simulink model "Jaco_3_7_IK"  (R2017a)
settings: Solver=VariableStepAuto  StartTime=0.0  StopTime=10.0  RelTol=1e-3  EnableMultiTasking=on
libraries: mblibv1 x42
settings Model: Creator=litia  LastModifiedBy=nathalie
settings OptimizationCC: LifeSpan=inf
settings DebuggingCC: SFUnexpectedBacktrackingDiag=warning  SFNoUnconditionalDefaultTransitionDiag=warning  SFExecutionAtInitializationDiag=none
settings GRTTargetCC: TargetLangStandard=C89/C90 (ANSI)
settings ConfigComp: CovMetricSettings=dw  CovHtmlReporting=on  CovSaveCumulativeToWorkspaceVar=on  CovSaveSingleToWorkspaceVar=on  CovExternalEMLEnable=off
settings SimMechanicsCC: VisOnUpdateDiagram=on  VisDuringSimulation=on

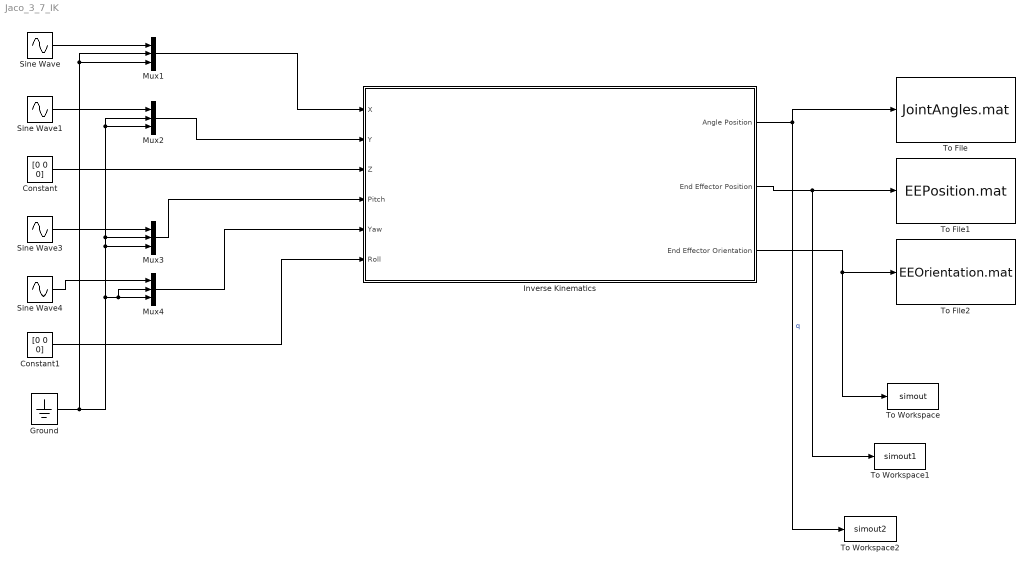
== system Jaco_3_7_IK ==
  Constant : Constant  Value=[0 0 0]  VectorParams1D=off
  Constant1 : Constant  Value=[0 0 0]  VectorParams1D=off
  Ground : Ground
  "Inverse Kinematics " : Subsystem
  Mux{1..4} (4 alike) : Mux  Inputs=3
  Sine Wave : Sin  Amplitude=0.2  Bias=-2  Frequency=2*pi  Phase=pi/2  SampleTime=0
  Sine Wave1 : Sin  Amplitude=0.2  Bias=-1  Frequency=2*pi  SampleTime=0
  Sine Wave3 : Sin  Amplitude=10  Bias=85  Frequency=2*pi  Phase=pi  SampleTime=0
  Sine Wave4 : Sin  Amplitude=10  Frequency=2*pi  Phase=pi/2  SampleTime=0
  To File : ToFile  Filename=JointAngles.mat  MatrixName=q  SaveFormat=Timeseries
  To File1 : ToFile  Filename=EEPosition.mat  MatrixName=xe  SaveFormat=Timeseries
  To File2 : ToFile  Filename=EEOrientation.mat  MatrixName=thetae  SaveFormat=Timeseries
  To Workspace : ToWorkspace  VariableName=simout  SaveFormat=Timeseries  SampleTime=-1
  To Workspace1 : ToWorkspace  VariableName=simout1  SaveFormat=Timeseries  SampleTime=-1
  To Workspace2 : ToWorkspace  VariableName=simout2  SaveFormat=Timeseries  SampleTime=-1
  wires:
  "Inverse Kinematics "/1("Angle Position ") -> To File/1, To Workspace2/1  "q"
  "Inverse Kinematics "/2(End Effector Position) -> To Workspace1/1, To File1/1
  "Inverse Kinematics "/3(End Effector Orientation) -> To Workspace/1, To File2/1
  Sine Wave/1 -> Mux1/1
  Sine Wave1/1 -> Mux2/1
  Ground/1 -> Mux1/3, Mux1/2, Mux3/3, Mux3/2, Mux2/3, Mux2/2, Mux4/2, Mux4/3
  Mux3/1 -> "Inverse Kinematics "/4(Pitch)
  Mux4/1 -> "Inverse Kinematics "/5(Yaw)
  Mux1/1 -> "Inverse Kinematics "/1(" X")
  Mux2/1 -> "Inverse Kinematics "/2(Y)
  Constant1/1 -> "Inverse Kinematics "/6("Roll ")
  Constant/1 -> "Inverse Kinematics "/3(Z)
  Sine Wave3/1 -> Mux3/1
  Sine Wave4/1 -> Mux4/1

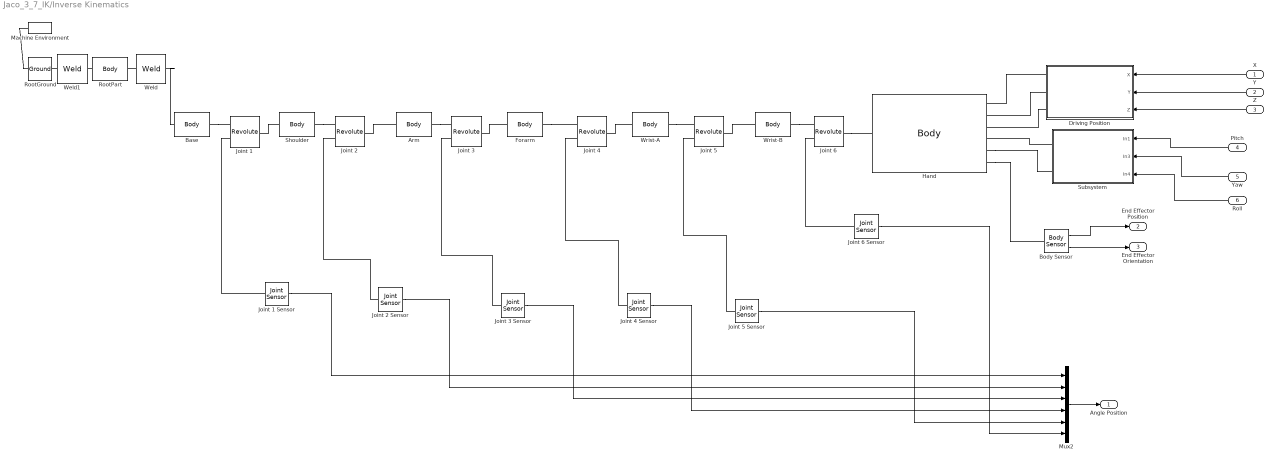
== system Jaco_3_7_IK/Inverse Kinematics  ==
  " X" : Inport
  Y : Inport  Port=2
  Z : Inport  Port=3
  Pitch : Inport  Port=4
  Yaw : Inport  Port=5
  "Roll " : Inport  Port=6
  Arm : mblibv1/Bodies/Body  LConnTagsString=CS2  RConnTagsString=CS3  UpdateFromCAD=on  DialogClass=MechanicalBodyBlock  Mass=1.056  MassUnits=kg  InertiaUnits=kg*m^2  Inertia=[0.0375645,-1.33324e-07,0.000108785;-1.33324e-07,0.0372402,-2.39225e-07;0.000108785,-2.39225e-07,0.00059301]  Shape=Cylinder  ShapeDims=[1 1]  ShapeUnits=m  ShapeUse=false  Density=1  DensityUnits=kg/m^3  DensityUse=false  GraphicsMode=GFXFILE  GraphicsFileName=Jaco_3_7 - arm_ass-1.STL  BodyColorSelMode=COLORPALETTE  BodyColor=[0.752941;0.752941;0.752941]  AttachedToCS=CS1  CG=Right$CG$[0.10282 0.0944444 0.508793]$WORLD$WORLD$m$[0.695251 0.715707 -0.0662524;0.718767 -0.692291 0.0640847;0 -0.092175 -0.995743]$3x3 Transform$rad$WORLD$false$none  WorkingFrames=Right$CS1$[-0.183907 0.105598 0.903425]$WORLD$WORLD$m$[0.695251 0.715707 -0.0662524;0.718767 -0.692291 0.0640847;0 -0.092175 -0.995743]$3x3 Transform$rad$WORLD$false$none#Left$CS2$[0.0767642 0.095252 0.300589]$WORLD$WORLD$m$[1 0 0;0 1 0;0 0 1]$3x3 Transform$rad$WORLD$true$none#Right$CS3$[0.10358 0.0686179 0.708843]$WORLD$WORLD$m$[1 0 0;0 1 0;0 0 1]$3x3 Transform$rad$WORLD$true$none  CGPos=[0.10282 0.0944444 0.508793]  CGRot=[0.695251 0.715707 -0.0662524;0.718767 -0.692291 0.0640847;0 -0.092175 -0.995743]  CS0Pos=[]  CS0Rot=[]  CS1Pos=[-0.183907 0.105598 0.903425]  CS1Rot=[0.695251 0.715707 -0.0662524;0.718767 -0.692291 0.0640847;0 -0.092175 -0.995743]  CS2Pos=[0.0767642 0.095252 0.300589]  CS2Rot=[1 0 0;0 1 0;0 0 1]  CS3Pos=[0.10358 0.0686179 0.708843]  CS3Rot=[1 0 0;0 1 0;0 0 1]  CS4Pos=[]  CS4Rot=[]  CS5Pos=[]  CS5Rot=[]  CS6Pos=[]  CS6Rot=[]  CS7Pos=[]  CS7Rot=[]  CS8Pos=[]  CS8Rot=[]  CS9Pos=[]  CS9Rot=[]  CS10Pos=[]  CS10Rot=[]  CS11Pos=[]  CS11Rot=[]  CS12Pos=[]  CS12Rot=[]  CS13Pos=[]  CS13Rot=[]  CS14Pos=[]  CS14Rot=[]  CS15Pos=[]  CS15Rot=[]  CS16Pos=[]  CS16Rot=[]  CS17Pos=[]  CS17Rot=[]  CS18Pos=[]  CS18Rot=[]  CS19Pos=[]  CS19Rot=[]  CS20Pos=[]  CS20Rot=[]
      settings: SourceProductName=Simscape Multibody  SourceProductBaseCode=MS
  Base : mblibv1/Bodies/Body  LConnTagsString=CS2  RConnTagsString=CS3  UpdateFromCAD=on  DialogClass=MechanicalBodyBlock  Mass=0.570939  MassUnits=kg  InertiaUnits=kg*m^2  Inertia=[0.00175947,1.92772e-07,-3.1782e-05;1.92772e-07,0.00176256,-3.18122e-05;-3.1782e-05,-3.18122e-05,0.000478232]  Shape=Cylinder  ShapeDims=[1 1]  ShapeUnits=m  ShapeUse=false  Density=1  DensityUnits=kg/m^3  DensityUse=false  GraphicsMode=GFXFILE  GraphicsFileName=Jaco_3_7 - base_ass-1.STL  BodyColorSelMode=COLORPALETTE  BodyColor=[0.752941;0.752941;0.752941]  AttachedToCS=CS1  CG=Right$CG$[0.0747134 0.093124 0.128067]$WORLD$WORLD$m$[1 0 0;0 1 0;0 0 1]$3x3 Transform$rad$WORLD$false$none  WorkingFrames=Right$CS1$[0.106448 0.0299726 -0.0762042]$WORLD$WORLD$m$[1 0 0;0 1 0;0 0 1]$3x3 Transform$rad$WORLD$false$none#Left$CS2$[0.0747134 0.093124 0.128067]$WORLD$WORLD$m$[1 0 0;0 1 0;0 0 1]$3x3 Transform$rad$WORLD$true$none#Right$CS3$[0.0753736 0.0938145 0.182089]$WORLD$WORLD$m$[1 0 0;0 1 0;0 0 1]$3x3 Transform$rad$WORLD$true$none  CGPos=[0.0747134 0.093124 0.128067]  CGRot=[1 0 0;0 1 0;0 0 1]  CS0Pos=[]  CS0Rot=[]  CS1Pos=[0.106448 0.0299726 -0.0762042]  CS1Rot=[1 0 0;0 1 0;0 0 1]  CS2Pos=[0.0747134 0.093124 0.128067]  CS2Rot=[1 0 0;0 1 0;0 0 1]  CS3Pos=[0.0753736 0.0938145 0.182089]  CS3Rot=[1 0 0;0 1 0;0 0 1]  CS4Pos=[]  CS4Rot=[]  CS5Pos=[]  CS5Rot=[]  CS6Pos=[]  CS6Rot=[]  CS7Pos=[]  CS7Rot=[]  CS8Pos=[]  CS8Rot=[]  CS9Pos=[]  CS9Rot=[]  CS10Pos=[]  CS10Rot=[]  CS11Pos=[]  CS11Rot=[]  CS12Pos=[]  CS12Rot=[]  CS13Pos=[]  CS13Rot=[]  CS14Pos=[]  CS14Rot=[]  CS15Pos=[]  CS15Rot=[]  CS16Pos=[]  CS16Rot=[]  CS17Pos=[]  CS17Rot=[]  CS18Pos=[]  CS18Rot=[]  CS19Pos=[]  CS19Rot=[]  CS20Pos=[]  CS20Rot=[]
      settings: SourceProductName=Simscape Multibody  SourceProductBaseCode=MS
  Body Sensor : mblibv1/Sensors &  Actuators/Body Sensor  UpdateFromCAD=off  PhysicalDomain=Mechanical  PortType=blob  Muxed=off  Pose=on  Angle=on  AngleUnits=deg  ArcVelocity=off  ArcVelocityUnits=deg/s  ArcAcceleration=off  ArcAccelerationUnits=deg/s^2  CoordPosition=on  CoordPositionUnits=m  Velocity=off  VelocityUnits=m/s  Acceleration=off  AccelerationUnits=m/s^2  Quaternion=on  QuaternionDT=off  QuaternionDDT=off  QuaternionUnits=off  OutputVector=[1]  ActiveIO=on  Width=12  DialogClass=MechanicalSensorBlock  ReferenceFrame=Absolute (World)
      settings: SourceProductName=Simscape Multibody  SourceProductBaseCode=MS
  Driving Position : Subsystem
  Forarm : mblibv1/Bodies/Body  LConnTagsString=CS2  RConnTagsString=CS3  UpdateFromCAD=on  DialogClass=MechanicalBodyBlock  Mass=0.735414  MassUnits=kg  InertiaUnits=kg*m^2  Inertia=[0.00626271,-0.000115651,1.81814e-08;-0.000115651,0.000377159,4.13244e-07;1.81814e-08,4.13244e-07,0.00610747]  Shape=Cylinder  ShapeDims=[1 1]  ShapeUnits=m  ShapeUse=false  Density=1  DensityUnits=kg/m^3  DensityUse=false  GraphicsMode=GFXFILE  GraphicsFileName=Jaco_3_7 - forarm_ass-1.STL  BodyColorSelMode=COLORPALETTE  BodyColor=[0.752941;0.752941;0.752941]  AttachedToCS=CS1  CG=Right$CG$[0.142291 0.0111153 0.740623]$WORLD$WORLD$m$[0.695251 0.650811 0.305076;0.718767 -0.629518 -0.295094;0 0.424443 -0.905455]$3x3 Transform$rad$WORLD$false$none  WorkingFrames=Right$CS1$[-0.0310579 0.0970807 0.899014]$WORLD$WORLD$m$[0.695251 0.650811 0.305076;0.718767 -0.629518 -0.295094;0 0.424443 -0.905455]$3x3 Transform$rad$WORLD$false$none#Left$CS2$[0.10358 0.0686179 0.708843]$WORLD$WORLD$m$[1 0 0;0 1 0;0 0 1]$3x3 Transform$rad$WORLD$true$none#Right$CS3$[0.230802 -0.0700932 0.796915]$WORLD$WORLD$m$[1 0 0;0 1 0;0 0 1]$3x3 Transform$rad$WORLD$true$none  CGPos=[0.142291 0.0111153 0.740623]  CGRot=[0.695251 0.650811 0.305076;0.718767 -0.629518 -0.295094;0 0.424443 -0.905455]  CS0Pos=[]  CS0Rot=[]  CS1Pos=[-0.0310579 0.0970807 0.899014]  CS1Rot=[0.695251 0.650811 0.305076;0.718767 -0.629518 -0.295094;0 0.424443 -0.905455]  CS2Pos=[0.10358 0.0686179 0.708843]  CS2Rot=[1 0 0;0 1 0;0 0 1]  CS3Pos=[0.230802 -0.0700932 0.796915]  CS3Rot=[1 0 0;0 1 0;0 0 1]  CS4Pos=[]  CS4Rot=[]  CS5Pos=[]  CS5Rot=[]  CS6Pos=[]  CS6Rot=[]  CS7Pos=[]  CS7Rot=[]  CS8Pos=[]  CS8Rot=[]  CS9Pos=[]  CS9Rot=[]  CS10Pos=[]  CS10Rot=[]  CS11Pos=[]  CS11Rot=[]  CS12Pos=[]  CS12Rot=[]  CS13Pos=[]  CS13Rot=[]  CS14Pos=[]  CS14Rot=[]  CS15Pos=[]  CS15Rot=[]  CS16Pos=[]  CS16Rot=[]  CS17Pos=[]  CS17Rot=[]  CS18Pos=[]  CS18Rot=[]  CS19Pos=[]  CS19Rot=[]  CS20Pos=[]  CS20Rot=[]
      settings: SourceProductName=Simscape Multibody  SourceProductBaseCode=MS
  Hand : mblibv1/Bodies/Body  LConnTagsString=CS2  RConnTagsString=CS3|CS4|CS5|CS6|CS7|CS8  UpdateFromCAD=on  DialogClass=MechanicalBodyBlock  Mass=0.395999  MassUnits=kg  InertiaUnits=kg*m^2  Inertia=[0.00124769,-0.000197969,-5.51354e-06;-0.000197969,0.000409818,-2.12169e-05;-5.51354e-06,-2.12169e-05,0.00139509]  Shape=Cylinder  ShapeDims=[1 1]  ShapeUnits=m  ShapeUse=false  Density=1  DensityUnits=kg/m^3  DensityUse=false  GraphicsMode=GFXFILE  GraphicsFileName=Jaco_3_7 - Hand_ass-1.STL  BodyColorSelMode=COLORPALETTE  BodyColor=[0.75294 0.75294 0.75294]  AttachedToCS=CS1  CG=Right$CG$[0.35442 -0.232757 0.799495]$WORLD$WORLD$m$[-0.439555 0.858973 -0.262597;-0.828489 -0.500657 -0.250895;-0.346983 0.107276 0.931716]$3x3 Transform$rad$WORLD$false$none  WorkingFrames=Right$CS1$[0.362295 -0.115327 0.65151]$WORLD$WORLD$m$[-0.439555 0.858973 -0.262597;-0.828489 -0.500657 -0.250895;-0.346983 0.107276 0.931716]$3x3 Transform$rad$WORLD$false$none#Left$CS2$[0.306767 -0.196631 0.795235]$WORLD$WORLD$m$[1 0 0;0 1 0;0 0 1]$3x3 Transform$rad$WORLD$true$none#Right$CS3$[0.306767 -0.196631 0.795235]$WORLD$WORLD$m$[1 0 0;0 1 0;0 0 1]$3x3 Transform$rad$WORLD$true$none#Right$CS4$[0.306767 -0.196631 0.795235]$WORLD$WORLD$m$[1 0 0;0 1 0;0 0 1]$3x3 Transform$rad$WORLD$true$none#Right$CS5$[0.306767 -0.196631 0.795235]$WORLD$WORLD$m$[1 0 0;0 1 0;0 0 1]$3x3 Transform$rad$WORLD$true$none#Right$CS6$[0.306767 -0.196631 0.795235]$WORLD$WORLD$m$[1 0 0;0 1 0;0 0 1]$3x3 Transform$rad$WORLD$true$none#Right$CS7$[0.306767 -0.196631 0.795235]$WORLD$WORLD$m$[1 0 0;0 1 0;0 0 1]$3x3 Transform$rad$WORLD$true$none#Right$CS8$[0.306767 -0.196631 0.795235]$WORLD$WORLD$m$[1 0 0;0 1 0;0 0 1]$3x3 Transform$rad$WORLD$true$none  CGPos=[0.35442 -0.232757 0.799495]  CGRot=[-0.439555 0.858973 -0.262597;-0.828489 -0.500657 -0.250895;-0.346983 0.107276 0.931716]  CS0Pos=[]  CS0Rot=[]  CS1Pos=[0.362295 -0.115327 0.65151]  CS1Rot=[-0.439555 0.858973 -0.262597;-0.828489 -0.500657 -0.250895;-0.346983 0.107276 0.931716]  CS2Pos=[0.306767 -0.196631 0.795235]  CS2Rot=[1 0 0;0 1 0;0 0 1]  CS3Pos=[0.306767 -0.196631 0.795235]  CS3Rot=[1 0 0;0 1 0;0 0 1]  CS4Pos=[0.306767 -0.196631 0.795235]  CS4Rot=[1 0 0;0 1 0;0 0 1]  CS5Pos=[0.306767 -0.196631 0.795235]  CS5Rot=[1 0 0;0 1 0;0 0 1]  CS6Pos=[0.306767 -0.196631 0.795235]  CS6Rot=[1 0 0;0 1 0;0 0 1]  CS7Pos=[0.306767 -0.196631 0.795235]  CS7Rot=[1 0 0;0 1 0;0 0 1]  CS8Pos=[0.306767 -0.196631 0.795235]  CS8Rot=[1 0 0;0 1 0;0 0 1]  CS9Pos=[]  CS9Rot=[]  CS10Pos=[]  CS10Rot=[]  CS11Pos=[]  CS11Rot=[]  CS12Pos=[]  CS12Rot=[]  CS13Pos=[]  CS13Rot=[]  CS14Pos=[]  CS14Rot=[]  CS15Pos=[]  CS15Rot=[]  CS16Pos=[]  CS16Rot=[]  CS17Pos=[]  CS17Rot=[]  CS18Pos=[]  CS18Rot=[]  CS19Pos=[]  CS19Rot=[]  CS20Pos=[]  CS20Rot=[]
      settings: SourceProductName=Simscape Multibody  SourceProductBaseCode=MS
  Joint 1 : mblibv1/Joints/Revolute  LConnTagsString=__newl0|SA1  RConnTagsString=__newr0  UpdateFromCAD=on  NumSAPorts=1  CutJoint=off  MarkAsCut=off  Primitives=prismatic  PrimitiveProps=R1$World$[0,0,1]$revolute  DialogClass=JointBlock  R1Axis=[0,0,1]
      settings: SourceProductName=Simscape Multibody  SourceProductBaseCode=MS
  Joint 1 Sensor : mblibv1/Sensors &  Actuators/Joint Sensor  UpdateFromCAD=off  PhysicalDomain=Mechanical  PortType=blob  Muxed=off  Pose=off  Angle=on  AngleUnits=deg  ArcVelocity=off  ArcVelocityUnits=deg/s  ArcAcceleration=off  ArcAccelerationUnits=deg/s^2  CoordPosition=on  CoordPositionUnits=m  Velocity=off  VelocityUnits=m/s  Acceleration=off  AccelerationUnits=m/s^2  Quaternion=on  QuaternionDT=off  QuaternionDDT=off  QuaternionUnits=off  OutputVector=[1]  ActiveIO=on  Width=1  DialogClass=MechanicalSensorBlock  Primitive=R1  Force=off  ForceUnits=N  Torque=off  TorqueUnits=N*m  ReferenceFrame=Absolute (World)  ReactionSensedSide=Base  ReactionReferenceFrame=Absolute (World)  ReactionForce=off  ReactionForceUnits=N  ReactionMoment=off  ReactionMomentUnits=N*m
      settings: SourceProductName=Simscape Multibody  SourceProductBaseCode=MS
  Joint 2 : mblibv1/Joints/Revolute  LConnTagsString=__newl0|SA1  RConnTagsString=__newr0  UpdateFromCAD=on  NumSAPorts=1  CutJoint=off  MarkAsCut=off  Primitives=prismatic  PrimitiveProps=R1$World$[0.695251,0.718767,0]$revolute  DialogClass=JointBlock  R1Axis=[0.695251,0.718767,0]
      settings: SourceProductName=Simscape Multibody  SourceProductBaseCode=MS
  Joint 2 Sensor : mblibv1/Sensors &  Actuators/Joint Sensor  UpdateFromCAD=off  PhysicalDomain=Mechanical  PortType=blob  Muxed=off  Pose=off  Angle=on  AngleUnits=deg  ArcVelocity=off  ArcVelocityUnits=deg/s  ArcAcceleration=off  ArcAccelerationUnits=deg/s^2  CoordPosition=on  CoordPositionUnits=m  Velocity=off  VelocityUnits=m/s  Acceleration=off  AccelerationUnits=m/s^2  Quaternion=on  QuaternionDT=off  QuaternionDDT=off  QuaternionUnits=off  OutputVector=[1]  ActiveIO=on  Width=1  DialogClass=MechanicalSensorBlock  Primitive=R1  Force=off  ForceUnits=N  Torque=off  TorqueUnits=N*m  ReferenceFrame=Absolute (World)  ReactionSensedSide=Base  ReactionReferenceFrame=Absolute (World)  ReactionForce=off  ReactionForceUnits=N  ReactionMoment=off  ReactionMomentUnits=N*m
      settings: SourceProductName=Simscape Multibody  SourceProductBaseCode=MS
  Joint 3 : mblibv1/Joints/Revolute  LConnTagsString=__newl0|SA1  RConnTagsString=__newr0  UpdateFromCAD=on  NumSAPorts=1  CutJoint=off  MarkAsCut=off  Primitives=prismatic  PrimitiveProps=R1$World$[-0.695251,-0.718767,0]$revolute  DialogClass=JointBlock  R1Axis=[-0.695251,-0.718767,0]
      settings: SourceProductName=Simscape Multibody  SourceProductBaseCode=MS
  Joint 3 Sensor : mblibv1/Sensors &  Actuators/Joint Sensor  UpdateFromCAD=off  PhysicalDomain=Mechanical  PortType=blob  Muxed=off  Pose=off  Angle=on  AngleUnits=deg  ArcVelocity=off  ArcVelocityUnits=deg/s  ArcAcceleration=off  ArcAccelerationUnits=deg/s^2  CoordPosition=on  CoordPositionUnits=m  Velocity=off  VelocityUnits=m/s  Acceleration=off  AccelerationUnits=m/s^2  Quaternion=on  QuaternionDT=off  QuaternionDDT=off  QuaternionUnits=off  OutputVector=[1]  ActiveIO=on  Width=1  DialogClass=MechanicalSensorBlock  Primitive=R1  Force=off  ForceUnits=N  Torque=off  TorqueUnits=N*m  ReferenceFrame=Absolute (World)  ReactionSensedSide=Base  ReactionReferenceFrame=Absolute (World)  ReactionForce=off  ReactionForceUnits=N  ReactionMoment=off  ReactionMomentUnits=N*m
      settings: SourceProductName=Simscape Multibody  SourceProductBaseCode=MS
  Joint 4 : mblibv1/Joints/Revolute  LConnTagsString=__newl0|SA1  RConnTagsString=__newr0  UpdateFromCAD=on  NumSAPorts=1  CutJoint=off  MarkAsCut=off  Primitives=prismatic  PrimitiveProps=R1$World$[0.650811,-0.629518,0.424443]$revolute  DialogClass=JointBlock  R1Axis=[0.650811,-0.629518,0.424443]
      settings: SourceProductName=Simscape Multibody  SourceProductBaseCode=MS
  Joint 4 Sensor : mblibv1/Sensors &  Actuators/Joint Sensor  UpdateFromCAD=off  PhysicalDomain=Mechanical  PortType=blob  Muxed=off  Pose=off  Angle=on  AngleUnits=deg  ArcVelocity=off  ArcVelocityUnits=deg/s  ArcAcceleration=off  ArcAccelerationUnits=deg/s^2  CoordPosition=on  CoordPositionUnits=m  Velocity=off  VelocityUnits=m/s  Acceleration=off  AccelerationUnits=m/s^2  Quaternion=on  QuaternionDT=off  QuaternionDDT=off  QuaternionUnits=off  OutputVector=[1]  ActiveIO=on  Width=1  DialogClass=MechanicalSensorBlock  Primitive=R1  Force=off  ForceUnits=N  Torque=off  TorqueUnits=N*m  ReferenceFrame=Absolute (World)  ReactionSensedSide=Base  ReactionReferenceFrame=Absolute (World)  ReactionForce=off  ReactionForceUnits=N  ReactionMoment=off  ReactionMomentUnits=N*m
      settings: SourceProductName=Simscape Multibody  SourceProductBaseCode=MS
  Joint 5 : mblibv1/Joints/Revolute  LConnTagsString=__newl0|SA1  RConnTagsString=__newr0  UpdateFromCAD=on  NumSAPorts=1  CutJoint=off  MarkAsCut=off  Primitives=prismatic  PrimitiveProps=R1$World$[0.15169,-0.946456,-0.284976]$revolute  DialogClass=JointBlock  R1Axis=[0.15169,-0.946456,-0.284976]
      settings: SourceProductName=Simscape Multibody  SourceProductBaseCode=MS
  Joint 5 Sensor : mblibv1/Sensors &  Actuators/Joint Sensor  UpdateFromCAD=off  PhysicalDomain=Mechanical  PortType=blob  Muxed=off  Pose=off  Angle=on  AngleUnits=deg  ArcVelocity=off  ArcVelocityUnits=deg/s  ArcAcceleration=off  ArcAccelerationUnits=deg/s^2  CoordPosition=on  CoordPositionUnits=m  Velocity=off  VelocityUnits=m/s  Acceleration=off  AccelerationUnits=m/s^2  Quaternion=on  QuaternionDT=off  QuaternionDDT=off  QuaternionUnits=off  OutputVector=[1]  ActiveIO=on  Width=1  DialogClass=MechanicalSensorBlock  Primitive=R1  Force=off  ForceUnits=N  Torque=off  TorqueUnits=N*m  ReferenceFrame=Absolute (World)  ReactionSensedSide=Base  ReactionReferenceFrame=Absolute (World)  ReactionForce=off  ReactionForceUnits=N  ReactionMoment=off  ReactionMomentUnits=N*m
      settings: SourceProductName=Simscape Multibody  SourceProductBaseCode=MS
  Joint 6 : mblibv1/Joints/Revolute  LConnTagsString=__newl0|SA1  RConnTagsString=__newr0  UpdateFromCAD=on  NumSAPorts=1  CutJoint=off  MarkAsCut=off  Primitives=prismatic  PrimitiveProps=R1$World$[0.858973,-0.500657,0.107276]$revolute  DialogClass=JointBlock  R1Axis=[0.858973,-0.500657,0.107276]
      settings: SourceProductName=Simscape Multibody  SourceProductBaseCode=MS
  Joint 6 Sensor : mblibv1/Sensors &  Actuators/Joint Sensor  UpdateFromCAD=off  PhysicalDomain=Mechanical  PortType=blob  Muxed=off  Pose=off  Angle=on  AngleUnits=deg  ArcVelocity=off  ArcVelocityUnits=deg/s  ArcAcceleration=off  ArcAccelerationUnits=deg/s^2  CoordPosition=on  CoordPositionUnits=m  Velocity=off  VelocityUnits=m/s  Acceleration=off  AccelerationUnits=m/s^2  Quaternion=on  QuaternionDT=off  QuaternionDDT=off  QuaternionUnits=off  OutputVector=[1]  ActiveIO=on  Width=1  DialogClass=MechanicalSensorBlock  Primitive=R1  Force=off  ForceUnits=N  Torque=off  TorqueUnits=N*m  ReferenceFrame=Absolute (World)  ReactionSensedSide=Base  ReactionReferenceFrame=Absolute (World)  ReactionForce=off  ReactionForceUnits=N  ReactionMoment=off  ReactionMomentUnits=N*m
      settings: SourceProductName=Simscape Multibody  SourceProductBaseCode=MS
  Machine Environment : mblibv1/Bodies/Machine Environment  PortType=env  PhysicalDomain=Mechanical  DialogTemplateClass=MECH.MachineEnvironment  SyncWhenCopied=off  Gravity=[0 0 -9.81]  GravityUnits=m/s^2  GravityAsSignal=off  Dimensionality=Auto-detect  AnalysisType=Kinematics  LinearAssemblyTolerance=1e-3  LinearAssemblyToleranceUnits=m  AngularAssemblyTolerance=1e-3  AngularAssemblyToleranceUnits=rad  ConstraintSolverType=Stabilizing  ConstraintRelTolerance=1e-4  ConstraintAbsTolerance=1e-4  UseRobustSingularityHandling=off  RedundancyAnalysisToleranceType=Automatically select tolerance  RedundancyAnalysisTolerance=1e-14  StatePerturbationType=Fixed  PerturbationSize=1e-5  VisualizeMachine=on  BodyVisualizationType=Use model default body geometries  BodyColorSelMode=Use model default  DefaultBodyColor=[1 0 0]
      settings: SourceProductName=Simscape Multibody  SourceProductBaseCode=MS
  Mux2 : Mux  Inputs=6
  RootGround : mblibv1/Bodies/Ground  UpdateFromCAD=on  LeftPortType=env  RightPortType=workingframe  PhysicalDomain=Mechanical  DialogClass=GroundBlock  CoordPosition=[0.154743,0.00421299,0.535333]  CoordPositionUnits=m  StateVectorMgrId=0  MachineId=[1 0]  ShowEnvPort=on  ParameterChecksum=[470875271, 2672832892, 1651714515, 3845969344]  TopologyChecksum=[674202019, 1973552515, 73634829, 3952998873]
      settings: SourceProductName=Simscape Multibody  SourceProductBaseCode=MS
  RootPart : mblibv1/Bodies/Body  LConnTagsString=CS3  RConnTagsString=CS2  UpdateFromCAD=on  DialogClass=MechanicalBodyBlock  Mass=0  MassUnits=kg  InertiaUnits=kg*m^2  Inertia=[0,0,0;0,0,0;0,0,0]  Shape=Cylinder  ShapeDims=[1 1]  ShapeUnits=m  ShapeUse=false  Density=1  DensityUnits=kg/m^3  DensityUse=false  GraphicsMode=MACHINE_DEFAULT  BodyColorSelMode=MACHINE_DEFAULT  BodyColor=[1;0;0]  AttachedToCS=CS1  CG=Right$CG$[0.154743 0.00421299 0.535333]$WORLD$WORLD$m$[1 0 0;0 1 0;0 0 1]$3x3 Transform$rad$WORLD$false$none  WorkingFrames=Right$CS1$[0 0 0]$WORLD$WORLD$m$[1 0 0;0 1 0;0 0 1]$3x3 Transform$rad$WORLD$false$none#Right$CS2$[0.0747134 0.093124 0.128067]$WORLD$WORLD$m$[1 0 0;0 1 0;0 0 1]$3x3 Transform$rad$WORLD$true$none#Left$CS3$[0.154743 0.00421299 0.535333]$WORLD$WORLD$m$[1 0 0;0 1 0;0 0 1]$3x3 Transform$rad$WORLD$true$none  CGPos=[0.154743 0.00421299 0.535333]  CGRot=[1 0 0;0 1 0;0 0 1]  CS0Pos=[]  CS0Rot=[]  CS1Pos=[0 0 0]  CS1Rot=[1 0 0;0 1 0;0 0 1]  CS2Pos=[0.0747134 0.093124 0.128067]  CS2Rot=[1 0 0;0 1 0;0 0 1]  CS3Pos=[0.154743 0.00421299 0.535333]  CS3Rot=[1 0 0;0 1 0;0 0 1]  CS4Pos=[]  CS4Rot=[]  CS5Pos=[]  CS5Rot=[]  CS6Pos=[]  CS6Rot=[]  CS7Pos=[]  CS7Rot=[]  CS8Pos=[]  CS8Rot=[]  CS9Pos=[]  CS9Rot=[]  CS10Pos=[]  CS10Rot=[]  CS11Pos=[]  CS11Rot=[]  CS12Pos=[]  CS12Rot=[]  CS13Pos=[]  CS13Rot=[]  CS14Pos=[]  CS14Rot=[]  CS15Pos=[]  CS15Rot=[]  CS16Pos=[]  CS16Rot=[]  CS17Pos=[]  CS17Rot=[]  CS18Pos=[]  CS18Rot=[]  CS19Pos=[]  CS19Rot=[]  CS20Pos=[]  CS20Rot=[]
      settings: SourceProductName=Simscape Multibody  SourceProductBaseCode=MS
  Shoulder : mblibv1/Bodies/Body  LConnTagsString=CS3  RConnTagsString=CS2  UpdateFromCAD=on  DialogClass=MechanicalBodyBlock  Mass=0.813994  MassUnits=kg  InertiaUnits=kg*m^2  Inertia=[0.0026546,0.000304923,5.38935e-08;0.000304923,0.000595598,-3.17242e-07;5.38935e-08,-3.17242e-07,0.00258406]  Shape=Cylinder  ShapeDims=[1 1]  ShapeUnits=m  ShapeUse=false  Density=1  DensityUnits=kg/m^3  DensityUse=false  GraphicsMode=GFXFILE  GraphicsFileName=Jaco_3_7 - shoulder_ass-1.STL  BodyColorSelMode=COLORPALETTE  BodyColor=[0.752941;0.752941;0.752941]  AttachedToCS=CS1  CG=Right$CG$[0.0698164 0.0880634 0.250193]$WORLD$WORLD$m$[0.695251 0 0.718767;0.718767 0 -0.695251;0 1 0]$3x3 Transform$rad$WORLD$false$none  WorkingFrames=Right$CS1$[-0.0564522 0.142463 0.184725]$WORLD$WORLD$m$[0.695251 0 0.718767;0.718767 0 -0.695251;0 1 0]$3x3 Transform$rad$WORLD$false$none#Right$CS2$[0.0767642 0.095252 0.300589]$WORLD$WORLD$m$[1 0 0;0 1 0;0 0 1]$3x3 Transform$rad$WORLD$true$none#Left$CS3$[0.0753736 0.0938145 0.182089]$WORLD$WORLD$m$[1 0 0;0 1 0;0 0 1]$3x3 Transform$rad$WORLD$true$none  CGPos=[0.0698164 0.0880634 0.250193]  CGRot=[0.695251 0 0.718767;0.718767 0 -0.695251;0 1 0]  CS0Pos=[]  CS0Rot=[]  CS1Pos=[-0.0564522 0.142463 0.184725]  CS1Rot=[0.695251 0 0.718767;0.718767 0 -0.695251;0 1 0]  CS2Pos=[0.0767642 0.095252 0.300589]  CS2Rot=[1 0 0;0 1 0;0 0 1]  CS3Pos=[0.0753736 0.0938145 0.182089]  CS3Rot=[1 0 0;0 1 0;0 0 1]  CS4Pos=[]  CS4Rot=[]  CS5Pos=[]  CS5Rot=[]  CS6Pos=[]  CS6Rot=[]  CS7Pos=[]  CS7Rot=[]  CS8Pos=[]  CS8Rot=[]  CS9Pos=[]  CS9Rot=[]  CS10Pos=[]  CS10Rot=[]  CS11Pos=[]  CS11Rot=[]  CS12Pos=[]  CS12Rot=[]  CS13Pos=[]  CS13Rot=[]  CS14Pos=[]  CS14Rot=[]  CS15Pos=[]  CS15Rot=[]  CS16Pos=[]  CS16Rot=[]  CS17Pos=[]  CS17Rot=[]  CS18Pos=[]  CS18Rot=[]  CS19Pos=[]  CS19Rot=[]  CS20Pos=[]  CS20Rot=[]
      settings: SourceProductName=Simscape Multibody  SourceProductBaseCode=MS
  Subsystem : Subsystem
  Weld : mblibv1/Joints/Weld  LConnTagsString=__newl0  RConnTagsString=__newr0  UpdateFromCAD=on  NumSAPorts=0  CutJoint=off  MarkAsCut=off  Primitives=weld  PrimitiveProps=W$WORLD$[0.57735,0.57735,0.57735]$weld  DialogClass=JointBlock  WAxis=[0.57735,0.57735,0.57735]
      settings: SourceProductName=Simscape Multibody  SourceProductBaseCode=MS
  Weld1 : mblibv1/Joints/Weld  LConnTagsString=__newl0  RConnTagsString=__newr0  UpdateFromCAD=on  NumSAPorts=0  CutJoint=off  MarkAsCut=off  Primitives=weld  PrimitiveProps=W$WORLD$[0.57735,0.57735,0.57735]$weld  DialogClass=JointBlock  WAxis=[0.57735,0.57735,0.57735]
      settings: SourceProductName=Simscape Multibody  SourceProductBaseCode=MS
  Wrist-A : mblibv1/Bodies/Body  LConnTagsString=CS3  RConnTagsString=CS2  UpdateFromCAD=on  DialogClass=MechanicalBodyBlock  Mass=0.44698  MassUnits=kg  InertiaUnits=kg*m^2  Inertia=[0.000407036,-3.06246e-08,5.0605e-09;-3.06246e-08,0.000239744,-8.7175e-05;5.0605e-09,-8.7175e-05,0.000376656]  Shape=Cylinder  ShapeDims=[1 1]  ShapeUnits=m  ShapeUse=false  Density=1  DensityUnits=kg/m^3  DensityUse=false  GraphicsMode=GFXFILE  GraphicsFileName=Jaco_3_7 - wrist1_ass-1.STL  BodyColorSelMode=COLORPALETTE  BodyColor=[0.752941;0.752941;0.752941]  AttachedToCS=CS1  CG=Right$CG$[0.251866 -0.101707 0.805258]$WORLD$WORLD$m$[0.709409 0.650811 -0.270524;0.30501 -0.629518 -0.714616;-0.63538 0.424443 -0.64509]$3x3 Transform$rad$WORLD$false$none  WorkingFrames=Right$CS1$[0.228148 -0.0304193 0.852839]$WORLD$WORLD$m$[0.709409 0.650811 -0.270524;0.30501 -0.629518 -0.714616;-0.63538 0.424443 -0.64509]$3x3 Transform$rad$WORLD$false$none#Right$CS2$[0.264276 -0.136155 0.802577]$WORLD$WORLD$m$[1 0 0;0 1 0;0 0 1]$3x3 Transform$rad$WORLD$true$none#Left$CS3$[0.230802 -0.0700932 0.796915]$WORLD$WORLD$m$[1 0 0;0 1 0;0 0 1]$3x3 Transform$rad$WORLD$true$none  CGPos=[0.251866 -0.101707 0.805258]  CGRot=[0.709409 0.650811 -0.270524;0.30501 -0.629518 -0.714616;-0.63538 0.424443 -0.64509]  CS0Pos=[]  CS0Rot=[]  CS1Pos=[0.228148 -0.0304193 0.852839]  CS1Rot=[0.709409 0.650811 -0.270524;0.30501 -0.629518 -0.714616;-0.63538 0.424443 -0.64509]  CS2Pos=[0.264276 -0.136155 0.802577]  CS2Rot=[1 0 0;0 1 0;0 0 1]  CS3Pos=[0.230802 -0.0700932 0.796915]  CS3Rot=[1 0 0;0 1 0;0 0 1]  CS4Pos=[]  CS4Rot=[]  CS5Pos=[]  CS5Rot=[]  CS6Pos=[]  CS6Rot=[]  CS7Pos=[]  CS7Rot=[]  CS8Pos=[]  CS8Rot=[]  CS9Pos=[]  CS9Rot=[]  CS10Pos=[]  CS10Rot=[]  CS11Pos=[]  CS11Rot=[]  CS12Pos=[]  CS12Rot=[]  CS13Pos=[]  CS13Rot=[]  CS14Pos=[]  CS14Rot=[]  CS15Pos=[]  CS15Rot=[]  CS16Pos=[]  CS16Rot=[]  CS17Pos=[]  CS17Rot=[]  CS18Pos=[]  CS18Rot=[]  CS19Pos=[]  CS19Rot=[]  CS20Pos=[]  CS20Rot=[]
      settings: SourceProductName=Simscape Multibody  SourceProductBaseCode=MS
  Wrist-B : mblibv1/Bodies/Body  LConnTagsString=CS3  RConnTagsString=CS2  UpdateFromCAD=on  DialogClass=MechanicalBodyBlock  Mass=0.44698  MassUnits=kg  InertiaUnits=kg*m^2  Inertia=[0.000407036,-3.06246e-08,5.0605e-09;-3.06246e-08,0.000239744,-8.7175e-05;5.0605e-09,-8.7175e-05,0.000376656]  Shape=Cylinder  ShapeDims=[1 1]  ShapeUnits=m  ShapeUse=false  Density=1  DensityUnits=kg/m^3  DensityUse=false  GraphicsMode=GFXFILE  GraphicsFileName=Jaco_3_7 - wrist2_ass-1.STL  BodyColorSelMode=COLORPALETTE  BodyColor=[0.752941;0.752941;0.752941]  AttachedToCS=CS1  CG=Right$CG$[0.28076 -0.170724 0.795794]$WORLD$WORLD$m$[-0.298122 0.15169 0.942398;-0.318695 -0.946456 0.0515257;0.899754 -0.284976 0.330502]$3x3 Transform$rad$WORLD$false$none  WorkingFrames=Right$CS1$[0.211333 -0.128563 0.759589]$WORLD$WORLD$m$[-0.298122 0.15169 0.942398;-0.318695 -0.946456 0.0515257;0.899754 -0.284976 0.330502]$3x3 Transform$rad$WORLD$false$none#Right$CS2$[0.306767 -0.196631 0.795235]$WORLD$WORLD$m$[1 0 0;0 1 0;0 0 1]$3x3 Transform$rad$WORLD$true$none#Left$CS3$[0.264276 -0.136155 0.802577]$WORLD$WORLD$m$[1 0 0;0 1 0;0 0 1]$3x3 Transform$rad$WORLD$true$none  CGPos=[0.28076 -0.170724 0.795794]  CGRot=[-0.298122 0.15169 0.942398;-0.318695 -0.946456 0.0515257;0.899754 -0.284976 0.330502]  CS0Pos=[]  CS0Rot=[]  CS1Pos=[0.211333 -0.128563 0.759589]  CS1Rot=[-0.298122 0.15169 0.942398;-0.318695 -0.946456 0.0515257;0.899754 -0.284976 0.330502]  CS2Pos=[0.306767 -0.196631 0.795235]  CS2Rot=[1 0 0;0 1 0;0 0 1]  CS3Pos=[0.264276 -0.136155 0.802577]  CS3Rot=[1 0 0;0 1 0;0 0 1]  CS4Pos=[]  CS4Rot=[]  CS5Pos=[]  CS5Rot=[]  CS6Pos=[]  CS6Rot=[]  CS7Pos=[]  CS7Rot=[]  CS8Pos=[]  CS8Rot=[]  CS9Pos=[]  CS9Rot=[]  CS10Pos=[]  CS10Rot=[]  CS11Pos=[]  CS11Rot=[]  CS12Pos=[]  CS12Rot=[]  CS13Pos=[]  CS13Rot=[]  CS14Pos=[]  CS14Rot=[]  CS15Pos=[]  CS15Rot=[]  CS16Pos=[]  CS16Rot=[]  CS17Pos=[]  CS17Rot=[]  CS18Pos=[]  CS18Rot=[]  CS19Pos=[]  CS19Rot=[]  CS20Pos=[]  CS20Rot=[]
      settings: SourceProductName=Simscape Multibody  SourceProductBaseCode=MS
  "Angle Position " : Outport
  End Effector Position : Outport  Port=2
  End Effector Orientation : Outport  Port=3
  wires:
  Joint 3 Sensor/1 -> Mux2/3
  Joint 6 Sensor/1 -> Mux2/6
  Mux2/1 -> "Angle Position "/1
  Joint 1 Sensor/1 -> Mux2/1
  Joint 2 Sensor/1 -> Mux2/2
  Joint 4 Sensor/1 -> Mux2/4
  Joint 5 Sensor/1 -> Mux2/5
  Z/1 -> Driving Position/3(Z)
  Body Sensor/1 -> End Effector Position/1
  Body Sensor/2 -> End Effector Orientation/1
  Yaw/1 -> Subsystem/2(In3)
  " X"/1 -> Driving Position/1("X ")
  Pitch/1 -> Subsystem/1(In1)
  "Roll "/1 -> Subsystem/3(In4)
  Y/1 -> Driving Position/2(Y)
  connections:
  Shoulder/RConn1 -- Joint 2/LConn1
  Joint 3 Sensor/LConn1 -- Joint 3/LConn2
  Weld/RConn1 -- Base/LConn1
  Joint 3/RConn1 -- Forarm/LConn1
  Joint 5/RConn1 -- Wrist-B/LConn1
  Joint 6/RConn1 -- Hand/LConn1
  Joint 6 Sensor/LConn1 -- Joint 6/LConn2
  Joint 2/RConn1 -- Arm/LConn1
  Joint 5 Sensor/LConn1 -- Joint 5/LConn2
  Joint 4 Sensor/LConn1 -- Joint 4/LConn2
  Arm/RConn1 -- Joint 3/LConn1
  Joint 1/RConn1 -- Shoulder/LConn1
  RootPart/RConn1 -- Weld/LConn1
  Base/RConn1 -- Joint 1/LConn1
  Wrist-A/RConn1 -- Joint 5/LConn1
  Wrist-B/RConn1 -- Joint 6/LConn1
  Weld1/RConn1 -- RootPart/LConn1
  Joint 4/RConn1 -- Wrist-A/LConn1
  Forarm/RConn1 -- Joint 4/LConn1
  Joint 2 Sensor/LConn1 -- Joint 2/LConn2
  RootGround/RConn1 -- Weld1/LConn1
  Machine Environment/RConn1 -- RootGround/LConn1
  Joint 1 Sensor/LConn1 -- Joint 1/LConn2
  Hand/RConn6 -- Body Sensor/LConn1
  Driving Position/RConn1 -- Hand/RConn1
  Driving Position/RConn2 -- Hand/RConn2
  Driving Position/RConn3 -- Hand/RConn3
  Subsystem/RConn1 -- Hand/RConn4
  Hand/RConn5 -- Subsystem/RConn2

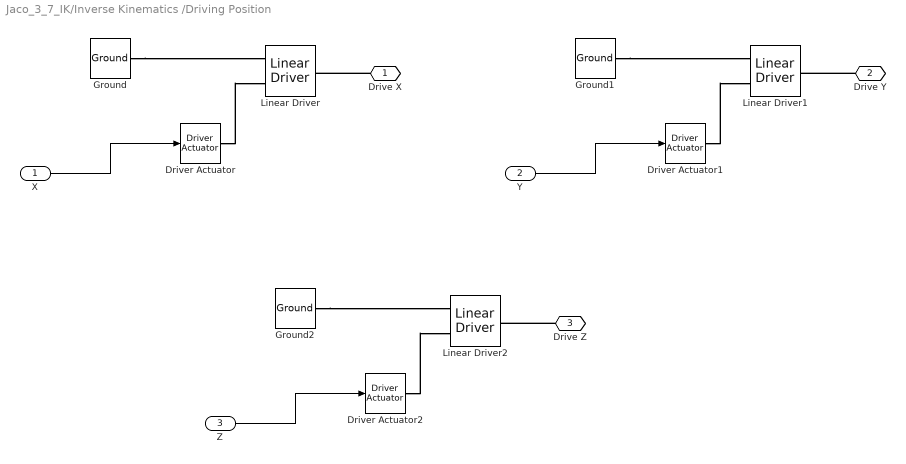
== system Jaco_3_7_IK/Inverse Kinematics /Driving Position ==
  "X " : Inport
  Y : Inport  Port=2
  Z : Inport  Port=3
  Driver Actuator : mblibv1/Sensors &  Actuators/Driver Actuator  UpdateFromCAD=off  PhysicalDomain=Mechanical  DialogClass=ConstraintActuatorBlock  PortType=blob  AngleUnits=deg  ArcVelocityUnits=deg/s  ArcAccelerationUnits=deg/s^2  CoordPositionUnits=m  VelocityUnits=m/s  AccelerationUnits=m/s^2  ActiveIO=on  Width=3
      settings: SourceProductName=Simscape Multibody  SourceProductBaseCode=MS
  Driver Actuator1 : mblibv1/Sensors &  Actuators/Driver Actuator  UpdateFromCAD=off  PhysicalDomain=Mechanical  DialogClass=ConstraintActuatorBlock  PortType=blob  AngleUnits=deg  ArcVelocityUnits=deg/s  ArcAccelerationUnits=deg/s^2  CoordPositionUnits=m  VelocityUnits=m/s  AccelerationUnits=m/s^2  ActiveIO=on  Width=3
      settings: SourceProductName=Simscape Multibody  SourceProductBaseCode=MS
  Driver Actuator2 : mblibv1/Sensors &  Actuators/Driver Actuator  UpdateFromCAD=off  PhysicalDomain=Mechanical  DialogClass=ConstraintActuatorBlock  PortType=blob  AngleUnits=deg  ArcVelocityUnits=deg/s  ArcAccelerationUnits=deg/s^2  CoordPositionUnits=m  VelocityUnits=m/s  AccelerationUnits=m/s^2  ActiveIO=on  Width=3
      settings: SourceProductName=Simscape Multibody  SourceProductBaseCode=MS
  Ground : mblibv1/Bodies/Ground  UpdateFromCAD=off  LeftPortType=env  RightPortType=workingframe  PhysicalDomain=Mechanical  DialogClass=GroundBlock  CoordPosition=[0 0 0]  CoordPositionUnits=m  StateVectorMgrId=-1  MachineId=[0 0]  ShowEnvPort=off  ParameterChecksum=[0 0 0 0]  TopologyChecksum=[0 0 0 0]
      settings: SourceProductName=Simscape Multibody  SourceProductBaseCode=MS
  Ground1 : mblibv1/Bodies/Ground  UpdateFromCAD=off  LeftPortType=env  RightPortType=workingframe  PhysicalDomain=Mechanical  DialogClass=GroundBlock  CoordPosition=[0 0 0]  CoordPositionUnits=m  StateVectorMgrId=-1  MachineId=[0 0]  ShowEnvPort=off  ParameterChecksum=[0 0 0 0]  TopologyChecksum=[0 0 0 0]
      settings: SourceProductName=Simscape Multibody  SourceProductBaseCode=MS
  Ground2 : mblibv1/Bodies/Ground  UpdateFromCAD=off  LeftPortType=env  RightPortType=workingframe  PhysicalDomain=Mechanical  DialogClass=GroundBlock  CoordPosition=[0 0 0]  CoordPositionUnits=m  StateVectorMgrId=-1  MachineId=[0 0]  ShowEnvPort=off  ParameterChecksum=[0 0 0 0]  TopologyChecksum=[0 0 0 0]
      settings: SourceProductName=Simscape Multibody  SourceProductBaseCode=MS
  Linear Driver : mblibv1/Constraints &  Drivers/Linear Driver  LConnTagsString=__newl0|SA1  RConnTagsString=__newr0  UpdateFromCAD=off  DialogClass=LinearDriverConstraint  NumSAPorts=1  GlobalCoordinate=X
      settings: SourceProductName=Simscape Multibody  SourceProductBaseCode=MS
  Linear Driver1 : mblibv1/Constraints &  Drivers/Linear Driver  LConnTagsString=__newl0|SA1  RConnTagsString=__newr0  UpdateFromCAD=off  DialogClass=LinearDriverConstraint  NumSAPorts=1  GlobalCoordinate=X
      settings: SourceProductName=Simscape Multibody  SourceProductBaseCode=MS
  Linear Driver2 : mblibv1/Constraints &  Drivers/Linear Driver  LConnTagsString=__newl0|SA1  RConnTagsString=__newr0  UpdateFromCAD=off  DialogClass=LinearDriverConstraint  NumSAPorts=1  GlobalCoordinate=X
      settings: SourceProductName=Simscape Multibody  SourceProductBaseCode=MS
  Drive X : PMIOPort  Port=1  Side=Right
  Drive Y : PMIOPort  Port=2  Side=Right
  Drive Z : PMIOPort  Port=3  Side=Right
  wires:
  "X "/1 -> Driver Actuator/1
  Y/1 -> Driver Actuator1/1
  Z/1 -> Driver Actuator2/1
  connections:
  Ground/RConn1 -- Linear Driver/LConn1
  Driver Actuator/RConn1 -- Linear Driver/LConn2
  Drive X/RConn1 -- Linear Driver/RConn1
  Drive Y/RConn1 -- Linear Driver1/RConn1
  Ground1/RConn1 -- Linear Driver1/LConn1
  Driver Actuator1/RConn1 -- Linear Driver1/LConn2
  Drive Z/RConn1 -- Linear Driver2/RConn1
  Ground2/RConn1 -- Linear Driver2/LConn1
  Driver Actuator2/RConn1 -- Linear Driver2/LConn2

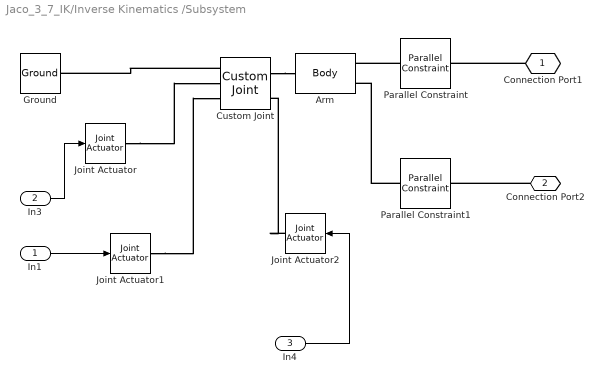
== system Jaco_3_7_IK/Inverse Kinematics /Subsystem ==
  In1 : Inport
  In3 : Inport  Port=2
  In4 : Inport  Port=3
  Arm : mblibv1/Bodies/Body  LConnTagsString=CS1  RConnTagsString=CS2|CS3  UpdateFromCAD=on  DialogClass=MechanicalBodyBlock  Mass=1.056  MassUnits=kg  InertiaUnits=kg*m^2  Inertia=[0.0375645,-1.33324e-07,0.000108785;-1.33324e-07,0.0372402,-2.39225e-07;0.000108785,-2.39225e-07,0.00059301]  Shape=Cylinder  ShapeDims=[1 1]  ShapeUnits=m  ShapeUse=false  Density=1  DensityUnits=kg/m^3  DensityUse=false  GraphicsMode=GFXFILE  GraphicsFileName=Jaco_3_7 - arm_ass-1.STL  BodyColorSelMode=COLORPALETTE  BodyColor=[0.75294 0.75294 0.75294]  AttachedToCS=CS1  CG=Right$CG$[0.10282 0.0944444 0.508793]$WORLD$WORLD$m$[0.695251 0.715707 -0.0662524;0.718767 -0.692291 0.0640847;0 -0.092175 -0.995743]$3x3 Transform$rad$WORLD$false$none  WorkingFrames=Left$CS1$[-0.183907 0.105598 0.903425]$WORLD$WORLD$m$[0.695251 0.715707 -0.0662524;0.718767 -0.692291 0.0640847;0 -0.092175 -0.995743]$3x3 Transform$rad$WORLD$true$none#Right$CS2$[0.0767642 0.095252 0.300589]$WORLD$WORLD$m$[1 0 0;0 1 0;0 0 1]$3x3 Transform$rad$WORLD$true$none#Right$CS3$[0.10358 0.0686179 0.708843]$WORLD$WORLD$m$[1 0 0;0 1 0;0 0 1]$3x3 Transform$rad$WORLD$true$none  CGPos=[0.10282 0.0944444 0.508793]  CGRot=[0.695251 0.715707 -0.0662524;0.718767 -0.692291 0.0640847;0 -0.092175 -0.995743]  CS0Pos=[]  CS0Rot=[]  CS1Pos=[-0.183907 0.105598 0.903425]  CS1Rot=[0.695251 0.715707 -0.0662524;0.718767 -0.692291 0.0640847;0 -0.092175 -0.995743]  CS2Pos=[0.0767642 0.095252 0.300589]  CS2Rot=[1 0 0;0 1 0;0 0 1]  CS3Pos=[0.10358 0.0686179 0.708843]  CS3Rot=[1 0 0;0 1 0;0 0 1]  CS4Pos=[]  CS4Rot=[]  CS5Pos=[]  CS5Rot=[]  CS6Pos=[]  CS6Rot=[]  CS7Pos=[]  CS7Rot=[]  CS8Pos=[]  CS8Rot=[]  CS9Pos=[]  CS9Rot=[]  CS10Pos=[]  CS10Rot=[]  CS11Pos=[]  CS11Rot=[]  CS12Pos=[]  CS12Rot=[]  CS13Pos=[]  CS13Rot=[]  CS14Pos=[]  CS14Rot=[]  CS15Pos=[]  CS15Rot=[]  CS16Pos=[]  CS16Rot=[]  CS17Pos=[]  CS17Rot=[]  CS18Pos=[]  CS18Rot=[]  CS19Pos=[]  CS19Rot=[]  CS20Pos=[]  CS20Rot=[]
      settings: SourceProductName=Simscape Multibody  SourceProductBaseCode=MS
  Custom Joint : mblibv1/Joints/Custom Joint  LConnTagsString=__newl0|SA1|SA2  RConnTagsString=__newr0|SA1  UpdateFromCAD=off  NumSAPorts=3  CutJoint=off  MarkAsCut=off  Primitives=prismatic  PrimitiveProps=R1$World$[1 0 0]$revolute#R2$World$[0 1 0]$Revolute#R3$World$[0 0 1]$Revolute  DialogClass=JointBlock  R1Axis=[1 0 0]  R2Axis=[0 1 0]  R3Axis=[0 0 1]  P1Axis=[]  P2Axis=[]  P3Axis=[]  SAxis=[]
      settings: SourceProductName=Simscape Multibody  SourceProductBaseCode=MS
  Ground : mblibv1/Bodies/Ground  UpdateFromCAD=off  LeftPortType=env  RightPortType=workingframe  PhysicalDomain=Mechanical  DialogClass=GroundBlock  CoordPosition=[-0.183907 0.105598 0.903425]  CoordPositionUnits=m  StateVectorMgrId=-1  MachineId=[0 0]  ShowEnvPort=off  ParameterChecksum=[0 0 0 0]  TopologyChecksum=[0 0 0 0]
      settings: SourceProductName=Simscape Multibody  SourceProductBaseCode=MS
  Joint Actuator : mblibv1/Sensors &  Actuators/Joint Actuator  UpdateFromCAD=off  PhysicalDomain=Mechanical  PortType=blob  ActuationStyle=Motion  AngleUnits=deg  ArcVelocityUnits=deg/s  ArcAccelerationUnits=deg/s^2  CoordPositionUnits=m  VelocityUnits=m/s  AccelerationUnits=m/s^2  ForceUnits=N  TorqueUnits=N*m  ActiveIO=on  Width=3  DialogClass=MechanicalActuatorBlock  Primitive=R2  ReferenceFrame=Absolute (World)
      settings: SourceProductName=Simscape Multibody  SourceProductBaseCode=MS
  Joint Actuator1 : mblibv1/Sensors &  Actuators/Joint Actuator  UpdateFromCAD=off  PhysicalDomain=Mechanical  PortType=blob  ActuationStyle=Motion  AngleUnits=deg  ArcVelocityUnits=deg/s  ArcAccelerationUnits=deg/s^2  CoordPositionUnits=m  VelocityUnits=m/s  AccelerationUnits=m/s^2  ForceUnits=N  TorqueUnits=N*m  ActiveIO=on  Width=3  DialogClass=MechanicalActuatorBlock  Primitive=R1  ReferenceFrame=Absolute (World)
      settings: SourceProductName=Simscape Multibody  SourceProductBaseCode=MS
  Joint Actuator2 : mblibv1/Sensors &  Actuators/Joint Actuator  UpdateFromCAD=off  PhysicalDomain=Mechanical  PortType=blob  ActuationStyle=Motion  AngleUnits=deg  ArcVelocityUnits=deg/s  ArcAccelerationUnits=deg/s^2  CoordPositionUnits=m  VelocityUnits=m/s  AccelerationUnits=m/s^2  ForceUnits=N  TorqueUnits=N*m  ActiveIO=on  Width=3  DialogClass=MechanicalActuatorBlock  Primitive=R3  ReferenceFrame=Absolute (World)
      settings: SourceProductName=Simscape Multibody  SourceProductBaseCode=MS
  Parallel Constraint : mblibv1/Constraints &  Drivers/Parallel Constraint  LConnTagsString=__newl0  RConnTagsString=__newr0  UpdateFromCAD=off  DialogClass=ParallelConstraint  NumSAPorts=0  Csys=WORLD  Axis=[1 0 0]
      settings: SourceProductName=Simscape Multibody  SourceProductBaseCode=MS
  Parallel Constraint1 : mblibv1/Constraints &  Drivers/Parallel Constraint  LConnTagsString=__newl0  RConnTagsString=__newr0  UpdateFromCAD=off  DialogClass=ParallelConstraint  NumSAPorts=0  Csys=WORLD  Axis=[1 0 0]
      settings: SourceProductName=Simscape Multibody  SourceProductBaseCode=MS
  Connection Port1 : PMIOPort  Port=1  Side=Right
  Connection Port2 : PMIOPort  Port=2  Side=Right
  wires:
  In4/1 -> Joint Actuator2/1
  In3/1 -> Joint Actuator/1
  In1/1 -> Joint Actuator1/1
  connections:
  Parallel Constraint1/LConn1 -- Arm/RConn2
  Parallel Constraint/LConn1 -- Arm/RConn1
  Custom Joint/RConn1 -- Arm/LConn1
  Custom Joint/LConn1 -- Ground/RConn1
  Joint Actuator/RConn1 -- Custom Joint/LConn2
  Joint Actuator2/RConn1 -- Custom Joint/RConn2
  Joint Actuator1/RConn1 -- Custom Joint/LConn3
  Connection Port1/RConn1 -- Parallel Constraint/RConn1
  Connection Port2/RConn1 -- Parallel Constraint1/RConn1
